simulink model "FloatingBall"  (R2024b)
settings: Solver=FixedStepAuto  StartTime=0.0  StopTime=inf  RelTol=1e-3  EnableMultiTasking=on
undefined symbols (not defined in the file or in its folder): Start
libraries: arduinolib x10, arduinoavrlib x2
(part 2 of 2)

== system FloatingBall/Motor Control/Previous Implementation/Switch Case Action Subsystem/Motor Pid/Differenzierer ==
  e : Inport
  Add : Sum
  Data Store Read : DataStoreRead  DataStoreName=Tf_motor  IndexOptions=Index vector (dialog)  Indices=1  OutputSizes=1
  Data Store Read1 : DataStoreRead  DataStoreName=T_s  IndexOptions=Index vector (dialog)  Indices=1  OutputSizes=1
  Data Store Read2 : DataStoreRead  DataStoreName=Kd_motor  IndexOptions=Index vector (dialog)  Indices=1  OutputSizes=1
  Divide : Product  Inputs=**/
  Divide1 : Product  Inputs=**/
  Sum : Sum  Inputs=|+-
  Sum1 : Sum  Inputs=|++
  Unit Delay : UnitDelay  SampleTime=0.02  HasFrameUpgradeWarning=on
  Unit Delay1 : UnitDelay  SampleTime=0.02  HasFrameUpgradeWarning=on
  d_k : Outport
  wires:
  Sum1/1 -> Unit Delay1/1, d_k/1  "d_k"
  Divide/1 -> Sum1/1
  e/1 -> Unit Delay/1, Sum/1
  Sum/1 -> Divide/2
  Unit Delay/1 -> Sum/2
  Divide1/1 -> Sum1/2
  Unit Delay1/1 -> Divide1/1  "d_k-1"
  Add/1 -> Divide1/3, Divide/3
  Data Store Read1/1 -> Add/1
  Data Store Read/1 -> Divide1/2, Add/2
  Data Store Read2/1 -> Divide/1

== system FloatingBall/Motor Control/Previous Implementation/Switch Case Action Subsystem/Motor Pid/Integrierer ==
  e : Inport
  Constant : Constant  Value=2
  Data Store Read : DataStoreRead  DataStoreName=Ki_motor  IndexOptions=Index vector (dialog)  Indices=1  OutputSizes=1
  Data Store Read1 : DataStoreRead  DataStoreName=T_s  IndexOptions=Index vector (dialog)  Indices=1  OutputSizes=1
  Divide : Product  Inputs=***/
  Sum : Sum  Inputs=|++
  Sum1 : Sum  Inputs=|++
  Unit Delay : UnitDelay  SampleTime=0.02  HasFrameUpgradeWarning=on
  Unit Delay1 : UnitDelay  SampleTime=0.02  HasFrameUpgradeWarning=on
  i_k : Outport
  wires:
  Divide/1 -> Unit Delay1/1, Sum1/1
  Sum/1 -> Divide/2
  e/1 -> Sum/1, Unit Delay/1
  Sum1/1 -> i_k/1
  Unit Delay1/1 -> Sum1/2
  Data Store Read1/1 -> Divide/3
  Unit Delay/1 -> Sum/2
  Data Store Read/1 -> Divide/1
  Constant/1 -> Divide/4

== system FloatingBall/Motor Control/Previous Implementation/Switch Case Action Subsystem/Motor Pid/Proportional-Glied ==
  e : Inport
  Data Store Read : DataStoreRead  DataStoreName=Kp_motor  IndexOptions=Index vector (dialog)  Indices=1  OutputSizes=1
  Product : Product
  p_k : Outport
  wires:
  Product/1 -> p_k/1  "p_k"
  e/1 -> Product/2
  Data Store Read/1 -> Product/1

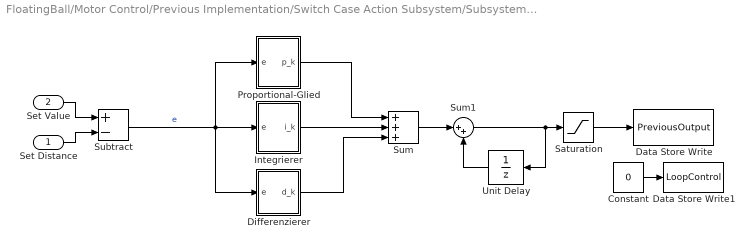
== system FloatingBall/Motor Control/Previous Implementation/Switch Case Action Subsystem/Subsystem/Pid ==
  Set Distance : Inport
  Set Value : Inport  Port=2
  Constant : Constant  Value=0
  Data Store Write : DataStoreWrite  DataStoreName=PreviousOutput  IndexOptions=Index vector (dialog)  Indices=1  OutputSizes=1
  Data Store Write1 : DataStoreWrite  DataStoreName=LoopControl  IndexOptions=Index vector (dialog)  Indices=1  OutputSizes=1
  Differenzierer : Subsystem
  Integrierer : Subsystem
  Proportional-Glied : Subsystem
  Saturation : Saturate  UpperLimit=3100  LowerLimit=0
  Subtract : Sum  Inputs=+-
  Sum : Sum  Inputs=+++
  Sum1 : Sum  Inputs=|++
  Unit Delay : UnitDelay  SampleTime=0.02  HasFrameUpgradeWarning=on
  wires:
  Integrierer/1(i_k) -> Sum/2
  Unit Delay/1 -> Sum1/2
  Sum1/1 -> Unit Delay/1, Saturation/1
  Proportional-Glied/1(p_k) -> Sum/1
  Set Value/1 -> Subtract/1
  Sum/1 -> Sum1/1
  Subtract/1 -> Integrierer/1(e), Differenzierer/1(e), Proportional-Glied/1(e)  "e"
  Differenzierer/1(d_k) -> Sum/3
  Saturation/1 -> Data Store Write/1
  Set Distance/1 -> Subtract/2
  Constant/1 -> Data Store Write1/1

== system FloatingBall/Motor Control/Subsystem/Cascaded Controller/Motor Pid/Differenzierer ==
  e : Inport
  Add : Sum
  Data Store Read : DataStoreRead  DataStoreName=Tf_motor  IndexOptions=Index vector (dialog)  Indices=1  OutputSizes=1
  Data Store Read1 : DataStoreRead  DataStoreName=T_s  IndexOptions=Index vector (dialog)  Indices=1  OutputSizes=1
  Data Store Read2 : DataStoreRead  DataStoreName=Kd_motor  IndexOptions=Index vector (dialog)  Indices=1  OutputSizes=1
  Divide : Product  Inputs=**/
  Divide1 : Product  Inputs=**/
  Sum : Sum  Inputs=|+-
  Sum1 : Sum  Inputs=|++
  Unit Delay : UnitDelay  SampleTime=0.02  HasFrameUpgradeWarning=on
  Unit Delay1 : UnitDelay  SampleTime=0.02  HasFrameUpgradeWarning=on
  d_k : Outport
  wires:
  Sum1/1 -> Unit Delay1/1, d_k/1  "d_k"
  Divide/1 -> Sum1/1
  e/1 -> Unit Delay/1, Sum/1
  Sum/1 -> Divide/2
  Unit Delay/1 -> Sum/2
  Divide1/1 -> Sum1/2
  Unit Delay1/1 -> Divide1/1  "d_k-1"
  Add/1 -> Divide1/3, Divide/3
  Data Store Read1/1 -> Add/1
  Data Store Read/1 -> Divide1/2, Add/2
  Data Store Read2/1 -> Divide/1

== system FloatingBall/Motor Control/Subsystem/Cascaded Controller/Motor Pid/Integrierer ==
  e : Inport
  Constant : Constant  Value=2
  Data Store Read : DataStoreRead  DataStoreName=Ki_motor  IndexOptions=Index vector (dialog)  Indices=1  OutputSizes=1
  Data Store Read1 : DataStoreRead  DataStoreName=T_s  IndexOptions=Index vector (dialog)  Indices=1  OutputSizes=1
  Divide : Product  Inputs=***/
  Sum : Sum  Inputs=|++
  Sum1 : Sum  Inputs=|++
  Unit Delay : UnitDelay  SampleTime=0.02  HasFrameUpgradeWarning=on
  Unit Delay1 : UnitDelay  SampleTime=0.02  HasFrameUpgradeWarning=on
  i_k : Outport
  wires:
  Divide/1 -> Unit Delay1/1, Sum1/1
  Sum/1 -> Divide/2
  e/1 -> Sum/1, Unit Delay/1
  Sum1/1 -> i_k/1
  Unit Delay1/1 -> Sum1/2
  Data Store Read1/1 -> Divide/3
  Unit Delay/1 -> Sum/2
  Data Store Read/1 -> Divide/1
  Constant/1 -> Divide/4

== system FloatingBall/Motor Control/Subsystem/Cascaded Controller/Motor Pid/Proportional-Glied ==
  e : Inport
  Data Store Read : DataStoreRead  DataStoreName=Kp_motor  IndexOptions=Index vector (dialog)  Indices=1  OutputSizes=1
  Product : Product
  p_k : Outport
  wires:
  Product/1 -> p_k/1  "p_k"
  e/1 -> Product/2
  Data Store Read/1 -> Product/1

== system FloatingBall/Motor Control/Subsystem/Cascaded Controller/Pid/Differenzierer ==
  e : Inport
  Add : Sum
  Data Store Read : DataStoreRead  DataStoreName=Tf_ctl  IndexOptions=Index vector (dialog)  Indices=1  OutputSizes=1
  Data Store Read1 : DataStoreRead  DataStoreName=T_s  IndexOptions=Index vector (dialog)  Indices=1  OutputSizes=1
  Data Store Read2 : DataStoreRead  DataStoreName=Kd_ctl  IndexOptions=Index vector (dialog)  Indices=1  OutputSizes=1
  Divide : Product  Inputs=**/
  Divide1 : Product  Inputs=**/
  Sum : Sum  Inputs=|+-
  Sum1 : Sum  Inputs=|++
  Unit Delay : UnitDelay  SampleTime=0.02  HasFrameUpgradeWarning=on
  Unit Delay1 : UnitDelay  SampleTime=0.02  HasFrameUpgradeWarning=on
  d_k : Outport
  wires:
  Sum1/1 -> Unit Delay1/1, d_k/1  "d_k"
  Divide/1 -> Sum1/1
  e/1 -> Unit Delay/1, Sum/1
  Sum/1 -> Divide/2
  Unit Delay/1 -> Sum/2
  Divide1/1 -> Sum1/2
  Unit Delay1/1 -> Divide1/1  "d_k-1"
  Add/1 -> Divide1/3, Divide/3
  Data Store Read1/1 -> Add/1
  Data Store Read/1 -> Divide1/2, Add/2
  Data Store Read2/1 -> Divide/1

== system FloatingBall/Motor Control/Subsystem/Cascaded Controller/Pid/Integrierer ==
  e : Inport
  Constant : Constant  Value=2
  Data Store Read : DataStoreRead  DataStoreName=Ki_ctl  IndexOptions=Index vector (dialog)  Indices=1  OutputSizes=1
  Data Store Read1 : DataStoreRead  DataStoreName=T_s  IndexOptions=Index vector (dialog)  Indices=1  OutputSizes=1
  Divide : Product  Inputs=***/
  Sum : Sum  Inputs=|++
  Sum1 : Sum  Inputs=|++
  Unit Delay : UnitDelay  SampleTime=0.02  HasFrameUpgradeWarning=on
  Unit Delay1 : UnitDelay  SampleTime=0.02  HasFrameUpgradeWarning=on
  i_k : Outport
  wires:
  Divide/1 -> Unit Delay1/1, Sum1/1
  Sum/1 -> Divide/2
  e/1 -> Sum/1, Unit Delay/1
  Sum1/1 -> i_k/1
  Unit Delay1/1 -> Sum1/2
  Data Store Read1/1 -> Divide/3
  Unit Delay/1 -> Sum/2
  Data Store Read/1 -> Divide/1
  Constant/1 -> Divide/4

== system FloatingBall/Motor Control/Subsystem/Cascaded Controller/Pid/Proportional-Glied ==
  e : Inport
  Data Store Read : DataStoreRead  DataStoreName=Kp_ctl  IndexOptions=Index vector (dialog)  Indices=1  OutputSizes=1
  Product : Product
  p_k : Outport
  wires:
  Product/1 -> p_k/1  "p_k"
  e/1 -> Product/2
  Data Store Read/1 -> Product/1

== system FloatingBall/Motor Control/Previous Implementation/Switch Case Action Subsystem/Subsystem/Pid/Differenzierer ==
  e : Inport
  Add : Sum
  Data Store Read : DataStoreRead  DataStoreName=Tf_ctl  IndexOptions=Index vector (dialog)  Indices=1  OutputSizes=1
  Data Store Read1 : DataStoreRead  DataStoreName=T_s  IndexOptions=Index vector (dialog)  Indices=1  OutputSizes=1
  Data Store Read2 : DataStoreRead  DataStoreName=Kd_ctl  IndexOptions=Index vector (dialog)  Indices=1  OutputSizes=1
  Divide : Product  Inputs=**/
  Divide1 : Product  Inputs=**/
  Sum : Sum  Inputs=|+-
  Sum1 : Sum  Inputs=|++
  Unit Delay : UnitDelay  SampleTime=0.02  HasFrameUpgradeWarning=on
  Unit Delay1 : UnitDelay  SampleTime=0.02  HasFrameUpgradeWarning=on
  d_k : Outport
  wires:
  Sum1/1 -> Unit Delay1/1, d_k/1  "d_k"
  Divide/1 -> Sum1/1
  e/1 -> Unit Delay/1, Sum/1
  Sum/1 -> Divide/2
  Unit Delay/1 -> Sum/2
  Divide1/1 -> Sum1/2
  Unit Delay1/1 -> Divide1/1  "d_k-1"
  Add/1 -> Divide1/3, Divide/3
  Data Store Read1/1 -> Add/1
  Data Store Read/1 -> Divide1/2, Add/2
  Data Store Read2/1 -> Divide/1

== system FloatingBall/Motor Control/Previous Implementation/Switch Case Action Subsystem/Subsystem/Pid/Integrierer ==
  e : Inport
  Constant : Constant  Value=2
  Data Store Read : DataStoreRead  DataStoreName=Ki_ctl  IndexOptions=Index vector (dialog)  Indices=1  OutputSizes=1
  Data Store Read1 : DataStoreRead  DataStoreName=T_s  IndexOptions=Index vector (dialog)  Indices=1  OutputSizes=1
  Divide : Product  Inputs=***/
  Sum : Sum  Inputs=|++
  Sum1 : Sum  Inputs=|++
  Unit Delay : UnitDelay  SampleTime=0.02  HasFrameUpgradeWarning=on
  Unit Delay1 : UnitDelay  SampleTime=0.02  HasFrameUpgradeWarning=on
  i_k : Outport
  wires:
  Divide/1 -> Unit Delay1/1, Sum1/1
  Sum/1 -> Divide/2
  e/1 -> Sum/1, Unit Delay/1
  Sum1/1 -> i_k/1
  Unit Delay1/1 -> Sum1/2
  Data Store Read1/1 -> Divide/3
  Unit Delay/1 -> Sum/2
  Data Store Read/1 -> Divide/1
  Constant/1 -> Divide/4

== system FloatingBall/Motor Control/Previous Implementation/Switch Case Action Subsystem/Subsystem/Pid/Proportional-Glied ==
  e : Inport
  Data Store Read : DataStoreRead  DataStoreName=Kp_ctl  IndexOptions=Index vector (dialog)  Indices=1  OutputSizes=1
  Product : Product
  p_k : Outport
  wires:
  Product/1 -> p_k/1  "p_k"
  e/1 -> Product/2
  Data Store Read/1 -> Product/1
